simulink model "PENDULOPID"  (R2022b)
settings: Solver=FixedStepAuto  StartTime=0.0  StopTime=100  FixedStep=0.001  RelTol=1e-3
undefined symbols (not defined in the file): b, b1, b2, beta, Fd, g, I2inv, ITinv, ITWinv, J, Kd, KdW, Ki, KiW, Kp, KpW, Kt, L, La, LW, MBAR, MP, Ra, rc
settings Model: Creator=mluser  LastModifiedBy=mluser

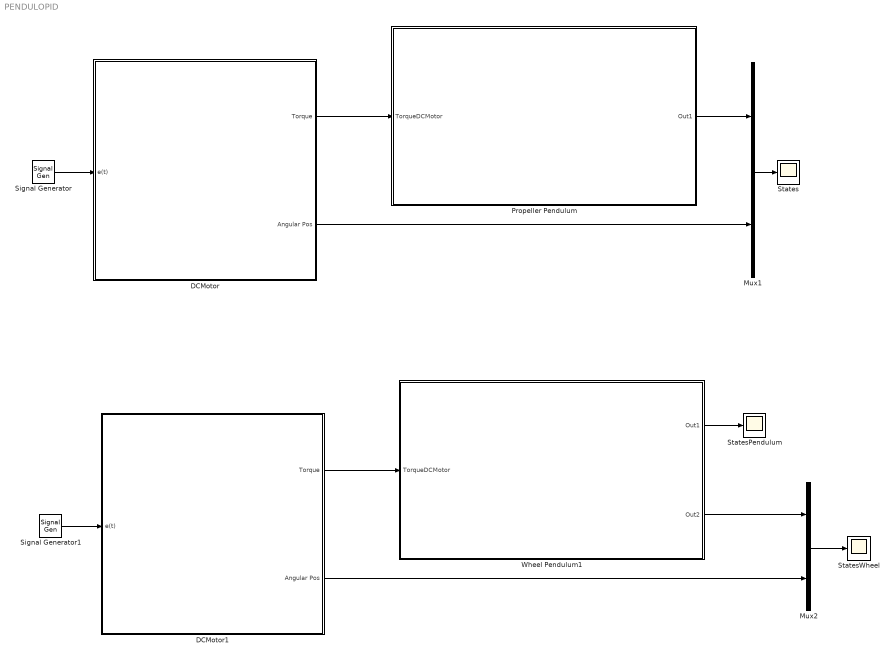
== system PENDULOPID ==
  DCMotor : Subsystem
  DCMotor1 : Subsystem
  Mux1 : Mux  Inputs=2
  Mux2 : Mux  Inputs=2
  Propeller Pendulum : Subsystem
  Signal Generator : SignalGenerator  Units=rad/sec
  Signal Generator1 : SignalGenerator  Units=rad/sec
  States : Scope
  StatesPendulum : Scope
  StatesWheel : Scope
  Wheel Pendulum1 : Subsystem
  wires:
  Signal Generator/1 -> DCMotor/1(e(t))
  DCMotor/1(Torque) -> Propeller Pendulum/1(TorqueDCMotor)
  DCMotor/2(Angular Pos) -> Mux1/2
  Propeller Pendulum/1(Out1) -> Mux1/1
  Mux1/1 -> States/1
  Mux2/1 -> StatesWheel/1
  DCMotor1/2(Angular Pos) -> Mux2/2
  Signal Generator1/1 -> DCMotor1/1(e(t))
  DCMotor1/1(Torque) -> Wheel Pendulum1/1(TorqueDCMotor)
  Wheel Pendulum1/2(Out2) -> Mux2/1
  Wheel Pendulum1/1(Out1) -> StatesPendulum/1

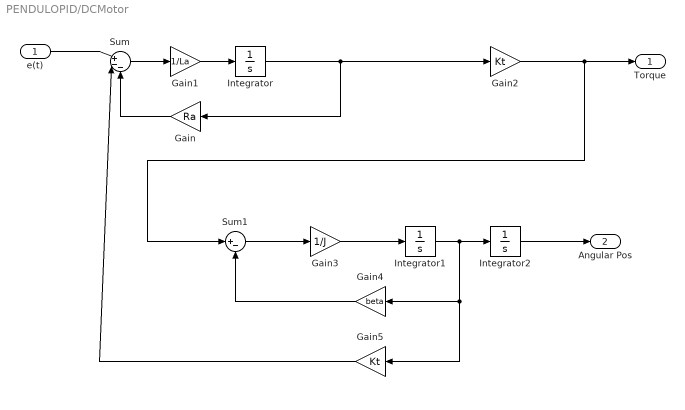
== system PENDULOPID/DCMotor ==
  e(t) : Inport
  Gain : Gain  Gain=Ra
  Gain1 : Gain  Gain=1/La
  Gain2 : Gain  Gain=Kt
  Gain3 : Gain  Gain=1/J
  Gain4 : Gain  Gain=beta
  Gain5 : Gain  Gain=Kt
  Integrator : Integrator
  Integrator1 : Integrator
  Integrator2 : Integrator
  Sum : Sum  Inputs=|+--
  Sum1 : Sum  Inputs=|+-
  Torque : Outport
  Angular Pos : Outport  Port=2
  wires:
  Integrator/1 -> Gain2/1, Gain/1
  Integrator1/1 -> Gain5/1, Gain4/1, Integrator2/1
  Integrator2/1 -> Angular Pos/1
  Gain3/1 -> Integrator1/1
  Sum1/1 -> Gain3/1
  Gain2/1 -> Torque/1, Sum1/1
  Gain4/1 -> Sum1/2
  Gain1/1 -> Integrator/1
  Sum/1 -> Gain1/1
  e(t)/1 -> Sum/1
  Gain/1 -> Sum/3
  Gain5/1 -> Sum/2

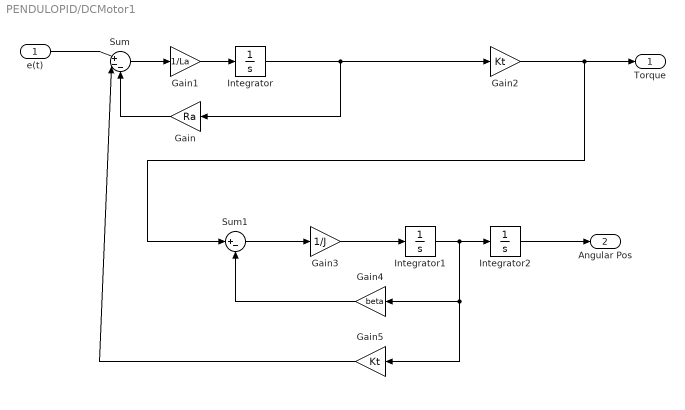
== system PENDULOPID/DCMotor1 ==
  e(t) : Inport
  Gain : Gain  Gain=Ra
  Gain1 : Gain  Gain=1/La
  Gain2 : Gain  Gain=Kt
  Gain3 : Gain  Gain=1/J
  Gain4 : Gain  Gain=beta
  Gain5 : Gain  Gain=Kt
  Integrator : Integrator
  Integrator1 : Integrator
  Integrator2 : Integrator
  Sum : Sum  Inputs=|+--
  Sum1 : Sum  Inputs=|+-
  Torque : Outport
  Angular Pos : Outport  Port=2
  wires:
  Integrator/1 -> Gain2/1, Gain/1
  Integrator1/1 -> Gain5/1, Gain4/1, Integrator2/1
  Integrator2/1 -> Angular Pos/1
  Gain3/1 -> Integrator1/1
  Sum1/1 -> Gain3/1
  Gain2/1 -> Torque/1, Sum1/1
  Gain4/1 -> Sum1/2
  Gain1/1 -> Integrator/1
  Sum/1 -> Gain1/1
  e(t)/1 -> Sum/1
  Gain/1 -> Sum/3
  Gain5/1 -> Sum/2

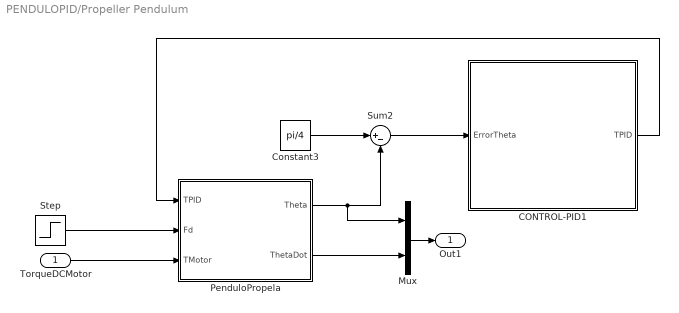
== system PENDULOPID/Propeller Pendulum ==
  TorqueDCMotor : Inport
  CONTROL-PID1 : Subsystem
  Constant3 : Constant  Value=pi/4
  Mux : Mux  Inputs=2
  PenduloPropela : Subsystem
  Step : Step  After=Fd  SampleTime=0
  Sum2 : Sum  Inputs=|+-
  Out1 : Outport
  wires:
  Constant3/1 -> Sum2/1
  PenduloPropela/1(Theta) -> Mux/1, Sum2/2
  PenduloPropela/2(ThetaDot) -> Mux/2
  TorqueDCMotor/1 -> PenduloPropela/3(TMotor)
  Mux/1 -> Out1/1
  Step/1 -> PenduloPropela/2(Fd)
  Sum2/1 -> CONTROL-PID1/1(ErrorTheta)
  CONTROL-PID1/1(TPID) -> PenduloPropela/1(TPID)

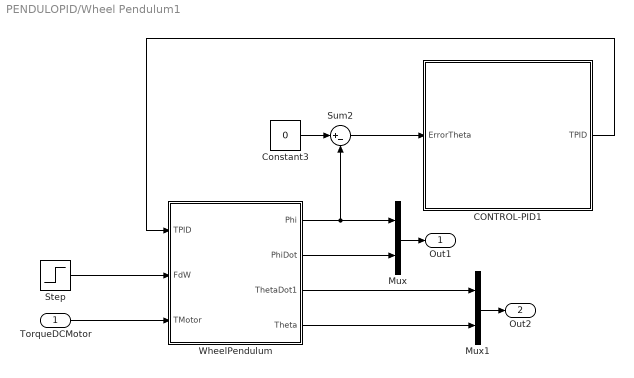
== system PENDULOPID/Wheel Pendulum1 ==
  TorqueDCMotor : Inport
  CONTROL-PID1 : Subsystem
  Constant3 : Constant  Value=0
  Mux : Mux  Inputs=2
  Mux1 : Mux  Inputs=2
  Step : Step  After=Fd  SampleTime=0
  Sum2 : Sum  Inputs=|+-
  WheelPendulum : Subsystem
  Out1 : Outport
  Out2 : Outport  Port=2
  wires:
  Constant3/1 -> Sum2/1
  WheelPendulum/1(Phi) -> Mux/1, Sum2/2
  WheelPendulum/2(PhiDot) -> Mux/2
  TorqueDCMotor/1 -> WheelPendulum/3(TMotor)
  Mux/1 -> Out1/1
  Step/1 -> WheelPendulum/2(FdW)
  Mux1/1 -> Out2/1
  WheelPendulum/3(ThetaDot1) -> Mux1/1
  WheelPendulum/4(Theta) -> Mux1/2
  Sum2/1 -> CONTROL-PID1/1(ErrorTheta)
  CONTROL-PID1/1(TPID) -> WheelPendulum/1(TPID)

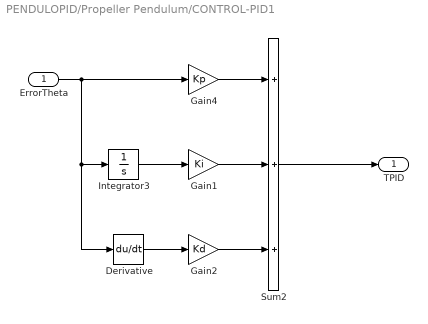
== system PENDULOPID/Propeller Pendulum/CONTROL-PID1 ==
  ErrorTheta : Inport
  Derivative : Derivative  CoefficientInTFapproximation=1/2.8915
  Gain1 : Gain  Gain=Ki
  Gain2 : Gain  Gain=Kd
  Gain4 : Gain  Gain=Kp
  Integrator3 : Integrator  InitialCondition=pi/2
  Sum2 : Sum  Inputs=+++
  TPID : Outport
  wires:
  ErrorTheta/1 -> Derivative/1, Integrator3/1, Gain4/1
  Integrator3/1 -> Gain1/1
  Sum2/1 -> TPID/1
  Derivative/1 -> Gain2/1
  Gain2/1 -> Sum2/3
  Gain1/1 -> Sum2/2
  Gain4/1 -> Sum2/1

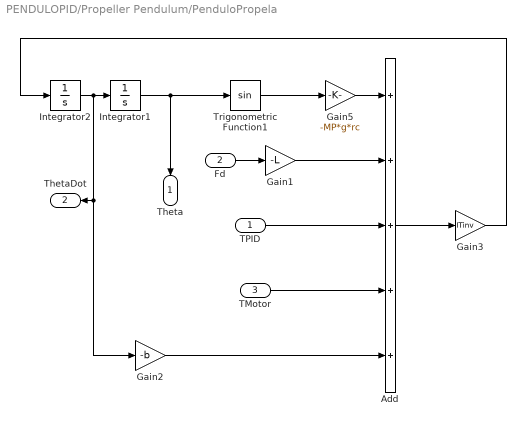
== system PENDULOPID/Propeller Pendulum/PenduloPropela ==
  TPID : Inport
  Fd : Inport  Port=2
  TMotor : Inport  Port=3
  Add : Sum  Inputs=+++++
  Gain1 : Gain  Gain=-L
  Gain2 : Gain  Gain=-b
  Gain3 : Gain  Gain=ITinv
  Gain5 : Gain  Gain=-MP*g*rc
  Integrator1 : Integrator  InitialCondition=pi/2
  Integrator2 : Integrator  InitialCondition=pi/2
  Trigonometric Function1 : Trigonometry
  Theta : Outport
  ThetaDot : Outport  Port=2
  wires:
  Integrator2/1 -> ThetaDot/1, Gain2/1, Integrator1/1
  Integrator1/1 -> Trigonometric Function1/1, Theta/1
  Add/1 -> Gain3/1
  Trigonometric Function1/1 -> Gain5/1
  Gain3/1 -> Integrator2/1
  Fd/1 -> Gain1/1
  Gain5/1 -> Add/1
  Gain1/1 -> Add/2
  TPID/1 -> Add/3
  TMotor/1 -> Add/4
  Gain2/1 -> Add/5

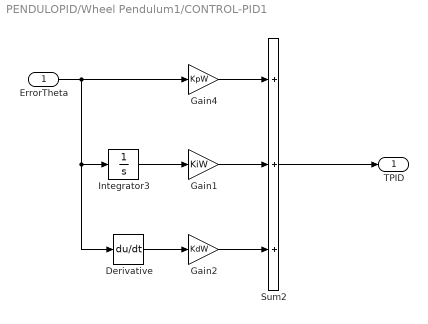
== system PENDULOPID/Wheel Pendulum1/CONTROL-PID1 ==
  ErrorTheta : Inport
  Derivative : Derivative  CoefficientInTFapproximation=1/2.7561
  Gain1 : Gain  Gain=KiW
  Gain2 : Gain  Gain=KdW
  Gain4 : Gain  Gain=KpW
  Integrator3 : Integrator  InitialCondition=pi/2
  Sum2 : Sum  Inputs=+++
  TPID : Outport
  wires:
  ErrorTheta/1 -> Derivative/1, Integrator3/1, Gain4/1
  Integrator3/1 -> Gain1/1
  Sum2/1 -> TPID/1
  Derivative/1 -> Gain2/1
  Gain2/1 -> Sum2/3
  Gain1/1 -> Sum2/2
  Gain4/1 -> Sum2/1

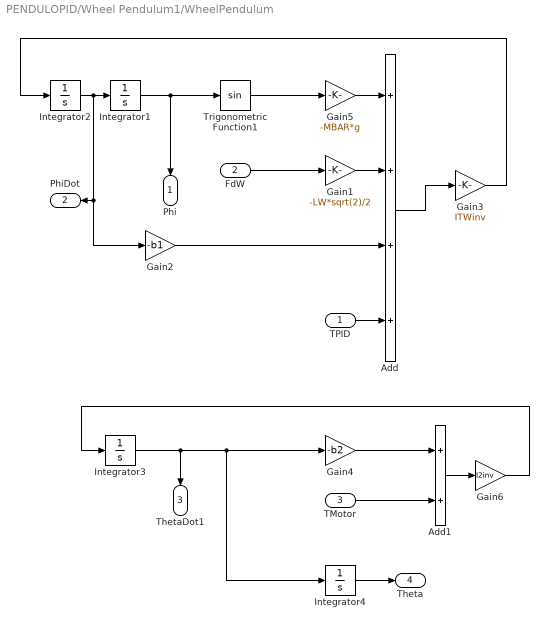
== system PENDULOPID/Wheel Pendulum1/WheelPendulum ==
  TPID : Inport
  FdW : Inport  Port=2
  TMotor : Inport  Port=3
  Add : Sum  Inputs=++++
  Add1 : Sum
  Gain1 : Gain  Gain=-LW*sqrt(2)/2
  Gain2 : Gain  Gain=-b1
  Gain3 : Gain  Gain=ITWinv
  Gain4 : Gain  Gain=-b2
  Gain5 : Gain  Gain=-MBAR*g
  Gain6 : Gain  Gain=I2inv
  Integrator{1..4} (4 alike) : Integrator  InitialCondition=pi/2
  Trigonometric Function1 : Trigonometry
  Phi : Outport
  PhiDot : Outport  Port=2
  ThetaDot1 : Outport  Port=3
  Theta : Outport  Port=4
  wires:
  Integrator2/1 -> PhiDot/1, Gain2/1, Integrator1/1
  Integrator1/1 -> Trigonometric Function1/1, Phi/1
  Add/1 -> Gain3/1
  Gain3/1 -> Integrator2/1
  FdW/1 -> Gain1/1
  Gain5/1 -> Add/1
  Gain1/1 -> Add/2
  Gain2/1 -> Add/3
  Gain4/1 -> Add1/1
  TMotor/1 -> Add1/2
  Add1/1 -> Gain6/1
  Gain6/1 -> Integrator3/1
  Integrator3/1 -> ThetaDot1/1, Integrator4/1, Gain4/1
  Integrator4/1 -> Theta/1
  Trigonometric Function1/1 -> Gain5/1
  TPID/1 -> Add/4
